simulink model "passeBas"  (R2019a)
settings: Solver=VariableStepAuto  StartTime=0.0  StopTime=10.0  RelTol=1e-3
undefined symbols (not defined in the file): fdesignblkfcn, gcbh
libraries: dspvision x1, Librairie x1
settings Model: Creator=shse  LastModifiedBy=shse

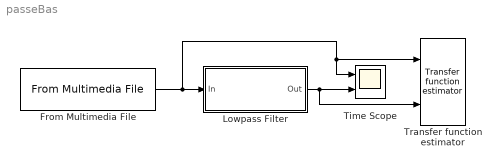
== system passeBas ==
  From Multimedia File : dspvision/From Multimedia File  inputFilename=C:\Users\shse\Nextcloud\L3\LU3EE105\Audio\Documents de TP et projet-20191118\Projet\guitare.wav  readRange=[1 Inf]  loop=on  numPlays=inf  outputStreams=Audio only  videoDataType=single  audioDataType=double  inheritSampleTime=on  userDefinedSampleTime=1/30  noAudioOutput=off  isIntensityVideo=off  fourcc=RGB  colorVideoFormat=Separate color signals  outputEOF=off  dataOrg=Column-major  audioFrameSize=1024  computeAudioFrameSize=off  outSamplingMode=Sample based
      settings: SourceProductName=DSP System Toolbox  SourceProductBaseCode=DS
  Lowpass Filter : Subsystem  DialogController=fdesignblkfcn  InitFcn=fdesignblkfcn(gcbh, {'InitFcn'});  mask(Lowpass Filter){}
      mask help: Design a lowpass filter
      settings: CopyFcn=fdesignblkfcn(gcbh, {'CopyFcn'});
      mask Help: helpview(mapfilelocation('dsp'), 'dsplowpassfilter');
      mask Display: disp('Lowpass')
  Time Scope : Scope  NumInputPorts=2
  Transfer function estimator : Librairie/Transfer function estimator  fee=11025  NN=1024
  wires:
  From Multimedia File/1 -> Time Scope/1, Transfer function estimator/1, Lowpass Filter/1(In)
  Lowpass Filter/1(Out) -> Transfer function estimator/2, Time Scope/2

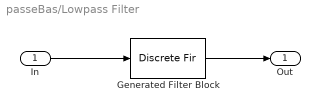
== system passeBas/Lowpass Filter ==
  In : Inport
  Generated Filter Block : DiscreteFir  Tag=BlockMethodSubSystem  Coefficients=[0.00287516122400231907 0.000852569555286751112 -0.00683152680924963614 -0.0205333876119196956 -0.0333395777943149771 -0.0345366506966156422 -0.0178048926385734468 0.0107453238059522487 0.0326142887392538161 0.0283717022959699382 -0.00560083946169475082 -0.0480059050987513905 -0.061222565688195299 -0.0153222833598335977 0.0878550951092589572 0.208858239917806443 0.290195572140625746 0.290195572140625746 0.208858239917806443 0.0878550951092589572 -0.0153222833598335977 -0.061222565688195299 -0.0480059050987513905 -0.00560083946169475082 0.0283717022959699382 0.0326142887392538161 0.0107453238059522487 -0.0178048926385734468 -0.0345366506966156422 -0.0333395777943149771 -0.0205333876119196956 -0.00683152680924963614 0.000852569555286751112 0.00287516122400231907]  InputProcessing=Columns as channels (frame based)
  Out : Outport
  wires:
  Generated Filter Block/1 -> Out/1
  In/1 -> Generated Filter Block/1
